simulink model "Seesaw_StateFB"  (R2024b)
settings: Solver=ode45  StartTime=0.0  StopTime=20  MaxStep=1e-3  RelTol=1e-4  AbsTol=1e-6
undefined symbols (not defined in the file): A_sw, B_sw, C_sw, D_sw, K_fb, V_sat
settings Model: Creator=Karim Negm  LastModifiedBy=Karim Negm

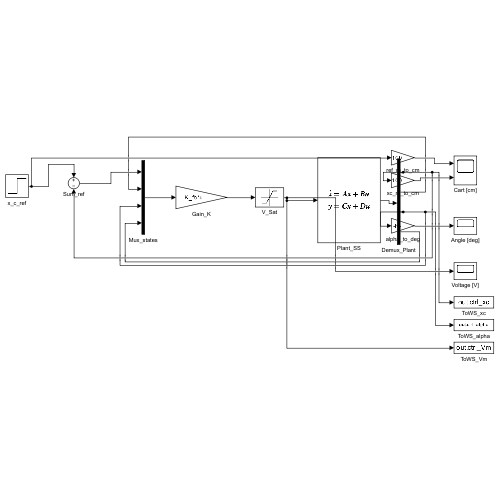
[thumbnail: Simulink's stored preview of the top-level diagram]
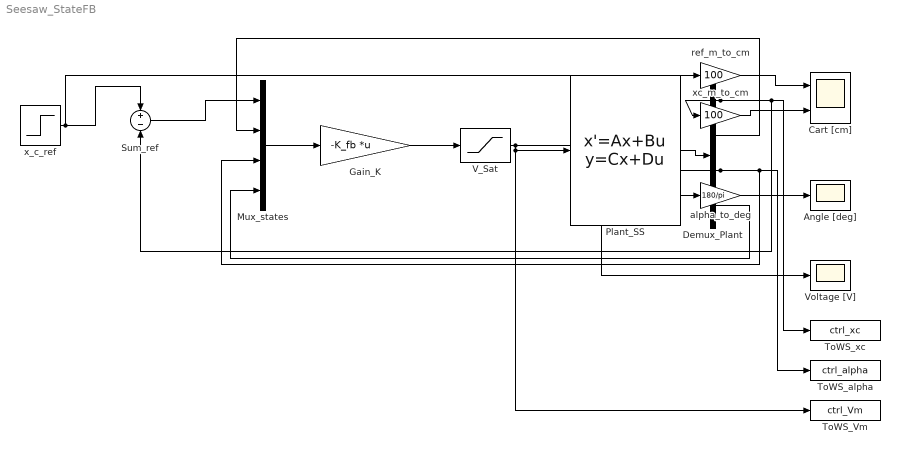
== system Seesaw_StateFB ==
  Angle [deg] : Scope
  Cart [cm] : Scope  NumInputPorts=2
  Demux_Plant : Demux
  Gain_K : Gain  Gain=-K_fb  Multiplication=Matrix(K*u)
  Mux_states : Mux
  Plant_SS : StateSpace  A=A_sw  B=B_sw  C=C_sw  D=D_sw  InitialCondition=[0; 0; 0.08; 0]
  Sum_ref : Sum  Inputs=+-
  ToWS_Vm : ToWorkspace  VariableName=ctrl_Vm  SaveFormat=Timeseries  SampleTime=-1
  ToWS_alpha : ToWorkspace  VariableName=ctrl_alpha  SaveFormat=Timeseries  SampleTime=-1
  ToWS_xc : ToWorkspace  VariableName=ctrl_xc  SaveFormat=Timeseries  SampleTime=-1
  V_Sat : Saturate  UpperLimit=V_sat  LowerLimit=-V_sat
  Voltage [V] : Scope
  alpha_to_deg : Gain  Gain=180/pi
  ref_m_to_cm : Gain  Gain=100
  x_c_ref : Step  Time=2  After=0  SampleTime=0
  xc_m_to_cm : Gain  Gain=100
  wires:
  x_c_ref/1 -> Sum_ref/1, ref_m_to_cm/1
  Sum_ref/1 -> Mux_states/1
  Mux_states/1 -> Gain_K/1
  Gain_K/1 -> V_Sat/1
  V_Sat/1 -> ToWS_Vm/1, Plant_SS/1, Voltage [V]/1
  ref_m_to_cm/1 -> Cart [cm]/1
  Plant_SS/1 -> Demux_Plant/1
  Demux_Plant/1 -> Sum_ref/2, ToWS_xc/1, xc_m_to_cm/1
  Demux_Plant/2 -> Mux_states/2
  Demux_Plant/3 -> Mux_states/3, ToWS_alpha/1, alpha_to_deg/1
  Demux_Plant/4 -> Mux_states/4
  xc_m_to_cm/1 -> Cart [cm]/2
  alpha_to_deg/1 -> Angle [deg]/1
